simulink model "sampleModel2025"  (R2023a)
settings: Solver=VariableStepAuto  StartTime=0.0  StopTime=10.0  RelTol=1e-3
libraries: hdlsllib x4, simulink x2
settings Model: Creator=user1  LastModifiedBy=user1

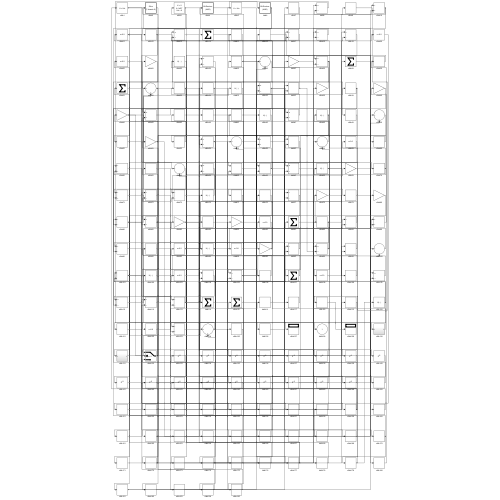
[thumbnail: Simulink's stored preview of the top-level diagram]
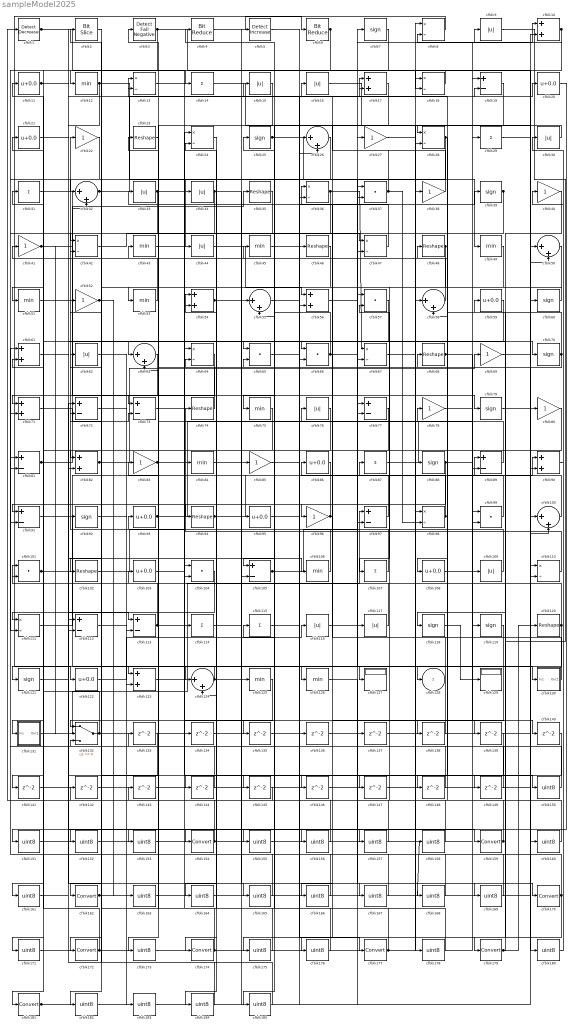
== system sampleModel2025 ==
  cfblk1 : simulink/Logic and Bit Operations/Detect Decrease  vinit=0.0  OutDataTypeStr=boolean
      settings: LibrarySourceBlock=|
      | hdlsllib/Logic and Bit
      | Operations/Detect
      | Decrease
  cfblk{10,17,54,56,61,71,82,90,123} (9 alike) : Sum
  cfblk{26,32,50,55,58,63,100,124} (8 alike) : Sum  Inputs=|++
  cfblk{37,57,65..66,99,101,104} (7 alike) : DotProduct  OutDataTypeStr=Inherit: Inherit via internal rule
  cfblk{23,35,46,48,68,74,94,102,120} (9 alike) : Reshape
  cfblk{11,20..21,59,86,93,95,103,108,122} (10 alike) : Bias  Bias=0.0  SaturateOnIntegerOverflow=off
  cfblk{19,72..73,77,81,89,91,97,105,112..113} (11 alike) : Sum  Inputs=+-
  cfblk{12,43,45,49,51,53,75,84,106,125..126} (11 alike) : MinMax
  cfblk{14,29,31,87,107,114..115} (7 alike) : Sum  Inputs=+
  cfblk{9,15..16,30,33..34,44,62,76,109,116..117} (12 alike) : Abs  SaturateOnIntegerOverflow=off
  cfblk{8,13,18,24,28,36,42,47,64,67,98,110..111} (13 alike) : Product  Inputs=*/  RndMeth=Zero  SaturateOnIntegerOverflow=on
  cfblk{7,25,39,60,70,79,88,92,118..119,121} (11 alike) : Signum
  cfblk127 : Display
  cfblk129 : Display
  cfblk130 : Subsystem
      settings: LibrarySourceBlock=|
      | hdlsllib/Ports &
      | Subsystems/Subsystem
  cfblk131 : Subsystem
      settings: LibrarySourceBlock=|
      | hdlsllib/Ports &
      | Subsystems/Subsystem
  cfblk132 : Switch  SaturateOnIntegerOverflow=off  InputSameDT=off
  cfblk{133..149} (17 alike) : Delay  SampleTime=1
  cfblk{150..153,155..158,160..161,163..169,171,173,175..176,178,180,182..185} (27 alike) : DataTypeConversion  OutDataTypeStr=uint8  SaturateOnIntegerOverflow=off  RndMeth=Floor
  cfblk{154,159,162,170,172,174,177,179,181} (9 alike) : DataTypeConversion  SaturateOnIntegerOverflow=off  RndMeth=Floor
  cfblk2 : hdlsllib/Logic and Bit Operations/Bit Slice  lidx=7  ridx=0
  cfblk{22,27,38,40..41,52,69,78,80,83,85,96} (12 alike) : Gain
  cfblk3 : hdlsllib/Logic and Bit Operations/Detect Fall Negative  vinit=0  OutDataTypeStr=boolean
  cfblk4 : hdlsllib/Logic and Bit Operations/Bit Reduce  mode=AND
  cfblk5 : simulink/Logic and Bit Operations/Detect Increase  vinit=0.0  OutDataTypeStr=boolean
      settings: LibrarySourceBlock=|
      | hdlsllib/Logic and Bit
      | Operations/Detect
      | Increase
  cfblk6 : hdlsllib/Logic and Bit Operations/Bit Reduce  mode=AND
  cfblk128 : Outport  VectorParamsAs1DForOutWhenUnconnected=off
  wires:
  cfblk32/1 -> cfblk17/1, cfblk82/1
  cfblk82/1 -> cfblk69/1, cfblk104/2
  cfblk100/1 -> cfblk66/1
  cfblk101/1 -> cfblk126/1, cfblk113/2
  cfblk8/1 -> cfblk122/1
  cfblk117/1 -> cfblk54/1
  cfblk120/1 -> cfblk101/1, cfblk65/2, cfblk141/1
  cfblk102/1 -> cfblk74/1
  cfblk24/1 -> cfblk174/1
  cfblk40/1 -> cfblk179/1
  cfblk80/1 -> cfblk181/1
  cfblk108/1 -> cfblk19/1
  cfblk41/1 -> cfblk63/1, cfblk132/2
  cfblk91/1 -> cfblk113/1
  cfblk81/1 -> cfblk35/1, cfblk145/1
  cfblk9/1 -> cfblk118/1
  cfblk31/1 -> cfblk79/1
  cfblk64/1 -> cfblk123/1
  cfblk44/1 -> cfblk56/1
  cfblk109/1 -> cfblk22/1
  cfblk131/1(Out1) -> cfblk97/1
  cfblk53/1 -> cfblk41/1
  cfblk118/1 -> cfblk129/1
  cfblk17/1 -> cfblk75/1
  cfblk111/1 -> cfblk89/1
  cfblk1/1 -> cfblk114/1, cfblk155/1
  cfblk62/1 -> cfblk123/2
  cfblk96/1 -> cfblk36/1, cfblk94/1
  cfblk36/1 -> cfblk67/1, cfblk81/2, cfblk128/1
  cfblk19/1 -> cfblk96/1
  cfblk52/1 -> cfblk2/1, cfblk163/1
  cfblk33/1 -> cfblk111/1, cfblk47/2
  cfblk56/1 -> cfblk9/1
  cfblk68/1 -> cfblk109/1, cfblk20/1
  cfblk16/1 -> cfblk100/1
  cfblk12/1 -> cfblk49/1, cfblk82/2
  cfblk130/1(Out1) -> cfblk86/1
  cfblk49/1 -> cfblk132/1
  cfblk46/1 -> cfblk154/1
  cfblk105/1 -> cfblk37/2, cfblk39/1
  cfblk23/1 -> cfblk73/1
  cfblk83/1 -> cfblk56/2, cfblk139/1
  cfblk95/1 -> cfblk78/1
  cfblk28/1 -> cfblk108/1, cfblk91/2, cfblk148/1
  cfblk122/1 -> cfblk116/1
  cfblk39/1 -> cfblk102/1, cfblk54/2
  cfblk97/1 -> cfblk87/1
  cfblk74/1 -> cfblk3/1
  cfblk27/1 -> cfblk170/1
  cfblk4/1 -> cfblk6/1
  cfblk3/1 -> cfblk51/1, cfblk60/1
  cfblk107/1 -> cfblk25/1
  cfblk14/1 -> cfblk110/1
  cfblk25/1 -> cfblk117/1, cfblk28/2
  cfblk89/1 -> cfblk43/1
  cfblk87/1 -> cfblk29/1
  cfblk65/1 -> cfblk36/2
  cfblk116/1 -> cfblk97/2
  cfblk132/1 -> cfblk89/2, cfblk42/2, cfblk92/1, cfblk31/1
  cfblk114/1 -> cfblk55/1
  cfblk103/1 -> cfblk90/1
  cfblk106/1 -> cfblk13/1
  cfblk58/1 -> cfblk21/1
  cfblk113/1 -> cfblk7/1, cfblk52/1, cfblk95/1
  cfblk47/1 -> cfblk23/1
  cfblk70/1 -> cfblk13/2, cfblk64/2
  cfblk115/1 -> cfblk177/1
  cfblk55/1 -> cfblk127/1
  cfblk18/1 -> cfblk12/1
  cfblk54/1 -> cfblk70/1, cfblk124/2
  cfblk11/1 -> cfblk19/2, cfblk65/1
  cfblk21/1 -> cfblk106/1
  cfblk30/1 -> cfblk28/1
  cfblk34/1 -> cfblk71/2, cfblk167/1
  cfblk93/1 -> cfblk26/1, cfblk10/2
  cfblk112/1 -> cfblk159/1
  cfblk79/1 -> cfblk90/2
  cfblk125/1 -> cfblk172/1
  cfblk10/1 -> cfblk8/2, cfblk18/2
  cfblk66/1 -> cfblk77/2, cfblk4/1
  cfblk99/1 -> cfblk48/1
  cfblk85/1 -> cfblk17/2
  cfblk124/1 -> cfblk121/1, cfblk146/1
  cfblk71/1 -> cfblk73/2
  cfblk2/1 -> cfblk32/1
  cfblk110/1 -> cfblk84/1
  cfblk90/1 -> cfblk30/1
  cfblk42/1 -> cfblk47/1
  cfblk38/1 -> cfblk15/1
  cfblk98/1 -> cfblk76/1, cfblk68/1
  cfblk94/1 -> cfblk26/2, cfblk124/1
  cfblk22/1 -> cfblk131/1(In1)
  cfblk60/1 -> cfblk53/1
  cfblk26/1 -> cfblk44/1
  cfblk51/1 -> cfblk32/2
  cfblk48/1 -> cfblk105/1, cfblk107/1
  cfblk84/1 -> cfblk130/1(In1)
  cfblk88/1 -> cfblk10/1, cfblk91/1
  cfblk37/1 -> cfblk16/1, cfblk98/2
  cfblk7/1 -> cfblk14/1
  cfblk6/1 -> cfblk42/1, cfblk111/2
  cfblk63/1 -> cfblk71/1
  cfblk50/1 -> cfblk162/1
  cfblk13/1 -> cfblk134/1
  cfblk134/1 -> cfblk58/1
  cfblk73/1 -> cfblk135/1
  cfblk135/1 -> cfblk77/1
  cfblk136/1 -> cfblk37/1
  cfblk137/1 -> cfblk110/2
  cfblk43/1 -> cfblk138/1
  cfblk138/1 -> cfblk8/1
  cfblk78/1 -> cfblk140/1
  cfblk141/1 -> cfblk105/2
  cfblk142/1 -> cfblk66/2
  cfblk143/1 -> cfblk67/2
  cfblk35/1 -> cfblk144/1
  cfblk144/1 -> cfblk81/1
  cfblk145/1 -> cfblk1/1
  cfblk146/1 -> cfblk100/2
  cfblk92/1 -> cfblk147/1
  cfblk147/1 -> cfblk18/1
  cfblk148/1 -> cfblk132/3
  cfblk123/1 -> cfblk149/1
  cfblk149/1 -> cfblk98/1
  cfblk5/1 -> cfblk150/1
  cfblk150/1 -> cfblk93/1
  cfblk20/1 -> cfblk151/1
  cfblk151/1 -> cfblk5/1
  cfblk133/1 -> cfblk152/1
  cfblk152/1 -> cfblk99/2
  cfblk15/1 -> cfblk153/1
  cfblk153/1 -> cfblk133/1
  cfblk154/1 -> cfblk64/1, cfblk99/1
  cfblk155/1 -> cfblk46/1
  cfblk57/1 -> cfblk156/1
  cfblk156/1 -> cfblk83/1
  cfblk121/1 -> cfblk157/1
  cfblk157/1 -> cfblk57/1
  cfblk158/1 -> cfblk57/2
  cfblk159/1 -> cfblk55/2, cfblk63/2, cfblk58/2
  cfblk69/1 -> cfblk160/1
  cfblk160/1 -> cfblk112/1
  cfblk104/1 -> cfblk161/1
  cfblk161/1 -> cfblk112/2
  cfblk162/1 -> cfblk158/1, cfblk34/1
  cfblk163/1 -> cfblk50/1
  cfblk139/1 -> cfblk164/1
  cfblk164/1 -> cfblk50/2
  cfblk61/1 -> cfblk165/1
  cfblk165/1 -> cfblk33/1
  cfblk119/1 -> cfblk166/1
  cfblk166/1 -> cfblk61/1
  cfblk167/1 -> cfblk61/2
  cfblk45/1 -> cfblk168/1
  cfblk168/1 -> cfblk104/1
  cfblk126/1 -> cfblk169/1
  cfblk169/1 -> cfblk45/1
  cfblk170/1 -> cfblk11/1, cfblk185/1
  cfblk59/1 -> cfblk171/1
  cfblk171/1 -> cfblk27/1
  cfblk172/1 -> cfblk101/2, cfblk62/1, cfblk119/1
  cfblk76/1 -> cfblk173/1
  cfblk173/1 -> cfblk125/1
  cfblk174/1 -> cfblk103/1, cfblk88/1, cfblk38/1
  cfblk77/1 -> cfblk175/1
  cfblk175/1 -> cfblk24/1
  cfblk140/1 -> cfblk176/1
  cfblk176/1 -> cfblk24/2
  cfblk177/1 -> cfblk143/1, cfblk142/1
  cfblk67/1 -> cfblk178/1
  cfblk178/1 -> cfblk115/1
  cfblk179/1 -> cfblk59/1, cfblk120/1
  cfblk29/1 -> cfblk180/1
  cfblk180/1 -> cfblk40/1
  cfblk181/1 -> cfblk137/1, cfblk85/1
  cfblk86/1 -> cfblk182/1
  cfblk182/1 -> cfblk80/1
  cfblk72/1 -> cfblk183/1
  cfblk183/1 -> cfblk136/1
  cfblk75/1 -> cfblk184/1
  cfblk184/1 -> cfblk72/1
  cfblk185/1 -> cfblk72/2

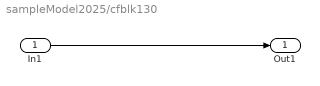
== system sampleModel2025/cfblk130 ==
  In1 : Inport
  Out1 : Outport
  wires:
  In1/1 -> Out1/1

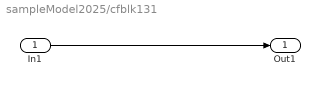
== system sampleModel2025/cfblk131 ==
  In1 : Inport
  Out1 : Outport
  wires:
  In1/1 -> Out1/1
